simulink model "propagatorGuz_jupiter"  (R2024b)
settings: Solver=FixedStepAuto  StartTime=0.0  StopTime=tf  FixedStep=3600  MaxStep=43200  MinStep=3600  RelTol=1e-8  AbsTol=1e-8
undefined symbols (not defined in the file or in its folder): area, burnOverride, initMass, mDot, ref, thrust, thrustingThreshold, thrustingThresholdMn
libraries: vrlib x5, simulink x4, matrix_library x4, aerolibsatdyn x1, aerolibutil x1
settings Model: Creator=miqui  LastModifiedBy=benit
settings SolverCC: InitialStep=3600
settings RTWCC: GPUComputeCapability=3.5

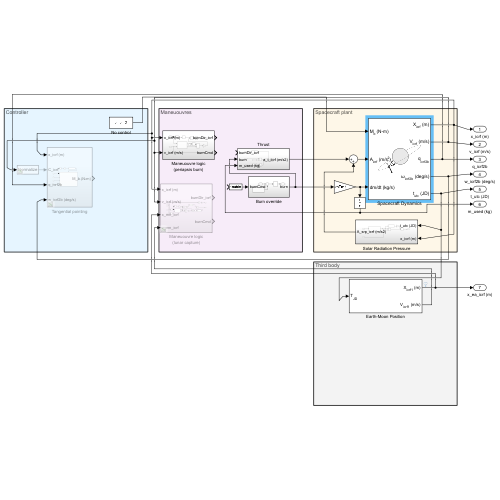
[thumbnail: Simulink's stored preview of the top-level diagram]
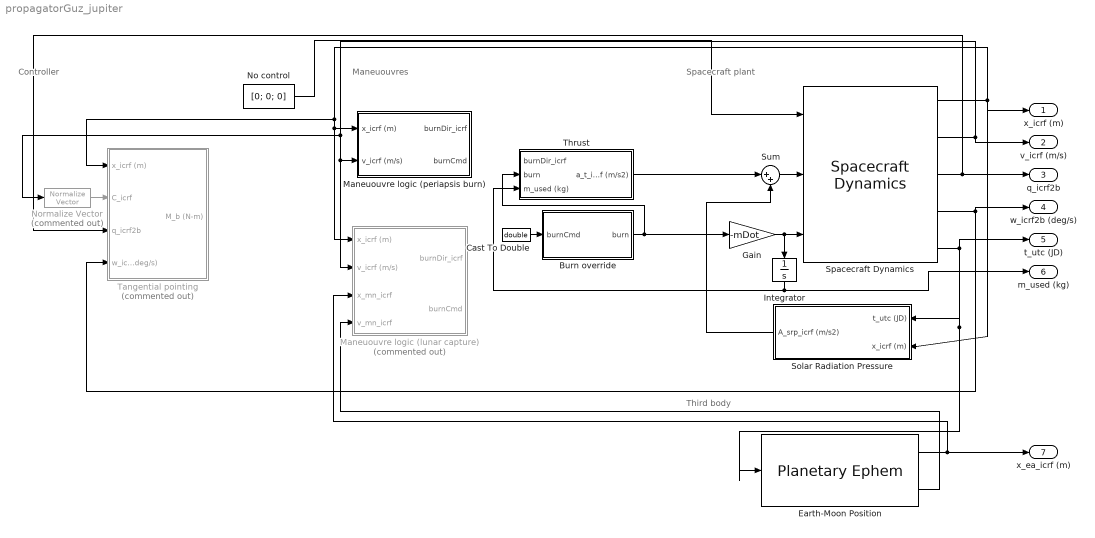
== system propagatorGuz_jupiter ==
  note: Third body
  note: Controller
  note: Maneuouvres
  note: Spacecraft plant
  Burn override : Subsystem
  Cast To Double : DataTypeConversion  OutDataTypeStr=double  SaturateOnIntegerOverflow=off  RndMeth=Floor
  Earth-Moon Position : PlanetaryEphem  units=m,m/s  center=Sun  target=Jupiter  useDateRange=on  startDate=startDate2  endDate=endDate
  Gain : Gain  Gain=-mDot
  Integrator : Integrator
  Maneuouvre logic (lunar capture) : Subsystem  Commented=on
  Maneuouvre logic (periapsis burn) : Subsystem
  No control : Constant  Value=[0; 0; 0]
  Normalize Vector : vrlib/Utilities/Normalize Vector  Commented=on  maxzero=0
  Solar Radiation Pressure : Subsystem
  Spacecraft Dynamics : SpacecraftDynamics  forcesIn=off  accelIn=on  startDate=startDate2  massType=Simple variable  mass=initMass  emptyMass=endMass  fullMass=initMass  inertia=[1, 0, 0; 0, 1, 0; 0, 0, 1]*initMass  outputFuelStatus=off  semiMajorAxis=sma  eccentricity=ecc  inclination=inc  raan=RAAN  argPeriapsis=aop  trueAnomaly=true_an  useGravGrad=off  centralBody=Sun  gravityModel=Point-mass  useEOPs=off  ephemerisStartDate=startDate2  ephemerisEndDate=endDate  useThirdBodyGravity=on  includeEarthGravity=off  includeMoonGravity=off  reflectivityCoeff=ref  srpArea=area
  Sum : Sum  Inputs=|++
  Tangential pointing : Subsystem  Commented=on
  Thrust : Subsystem
  x_icrf (m) : Outport
  v_icrf (m/s) : Outport  Port=2
  q_icrf2b : Outport  Port=3
  w_icrf2b (deg/s) : Outport  Port=4
  t_utc (JD) : Outport  Port=5
  m_used (kg) : Outport  Port=6
  x_ea_icrf (m) : Outport  Port=7
  wires:
  Spacecraft Dynamics/1 -> Maneuouvre logic (lunar capture)/1(x_icrf (m)), Maneuouvre logic (periapsis burn)/1(x_icrf (m)), Tangential pointing/1(x_icrf (m)), Solar Radiation Pressure/2(x_icrf (m)), x_icrf (m)/1
  Spacecraft Dynamics/2 -> Maneuouvre logic (lunar capture)/2(v_icrf (m/s)), Maneuouvre logic (periapsis burn)/2(v_icrf (m/s)), Normalize Vector/1, v_icrf (m/s)/1
  Spacecraft Dynamics/3 -> Tangential pointing/3(q_icrf2b), q_icrf2b/1
  Spacecraft Dynamics/4 -> Tangential pointing/4(w_icrf2b (deg/s)), w_icrf2b (deg/s)/1
  Spacecraft Dynamics/5 -> Earth-Moon Position/1, Solar Radiation Pressure/1(t_utc (JD)), t_utc (JD)/1
  Integrator/1 -> Thrust/3(m_used (kg)), m_used (kg)/1
  Gain/1 -> Spacecraft Dynamics/3, Integrator/1
  Sum/1 -> Spacecraft Dynamics/2
  Cast To Double/1 -> Burn override/1(burnCmd)
  Burn override/1(burn) -> Thrust/2(burn), Gain/1
  Thrust/1(a_t_icrf (m/s2)) -> Sum/1
  Earth-Moon Position/1 -> Maneuouvre logic (lunar capture)/3(x_mn_icrf), x_ea_icrf (m)/1
  Earth-Moon Position/2 -> Maneuouvre logic (lunar capture)/4(v_mn_icrf)
  Normalize Vector/1 -> Tangential pointing/2(C_icrf)
  No control/1 -> Spacecraft Dynamics/1
  Solar Radiation Pressure/1(A_srp_icrf (m/s2)) -> Sum/2

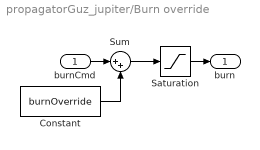
== system propagatorGuz_jupiter/Burn override ==
  burnCmd : Inport
  Constant : Constant  Value=burnOverride
  Saturation : Saturate  UpperLimit=1  LowerLimit=0
  Sum : Sum  Inputs=|++
  burn : Outport
  wires:
  Constant/1 -> Sum/2
  Saturation/1 -> burn/1
  burnCmd/1 -> Sum/1
  Sum/1 -> Saturation/1

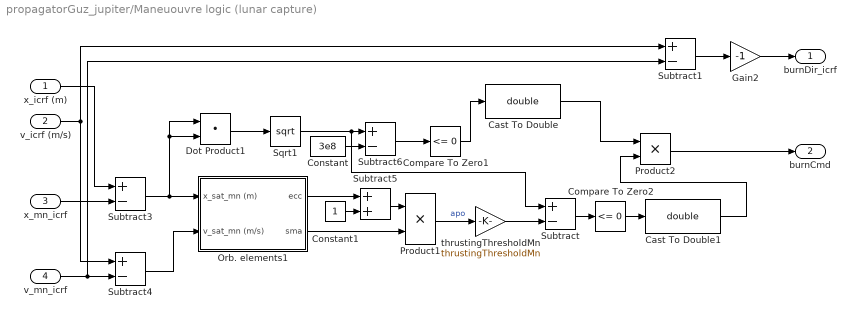
== system propagatorGuz_jupiter/Maneuouvre logic (lunar capture) ==
  x_icrf (m) : Inport
  v_icrf (m/s) : Inport  Port=2
  x_mn_icrf : Inport  Port=3
  v_mn_icrf : Inport  Port=4
  Cast To Double : DataTypeConversion  OutDataTypeStr=double  SaturateOnIntegerOverflow=off  RndMeth=Floor
  Cast To Double1 : DataTypeConversion  OutDataTypeStr=double  SaturateOnIntegerOverflow=off  RndMeth=Floor
  Compare To Zero1 : simulink/Logic and Bit Operations/Compare To Zero  relop=<=  OutDataTypeStr=boolean
  Compare To Zero2 : simulink/Logic and Bit Operations/Compare To Zero  relop=<=  OutDataTypeStr=boolean
  Constant : Constant  Value=3e8
  Constant1 : Constant
  Dot Product1 : DotProduct  OutDataTypeStr=Inherit: Inherit via internal rule
  Gain2 : Gain  Gain=-1
  Orb. elements1 : Subsystem
  Product1 : Product
  Product2 : Product
  Sqrt1 : Sqrt
  Subtract{,1,3..4,6} (5 alike) : Sum  Inputs=+-
  Subtract5 : Sum
  thrustingThresholdMn : Gain  Gain=thrustingThresholdMn
  burnDir_icrf : Outport
  burnCmd : Outport  Port=2
  wires:
  x_icrf (m)/1 -> Subtract3/1
  v_icrf (m/s)/1 -> Subtract1/1, Subtract4/1
  x_mn_icrf/1 -> Subtract3/2
  v_mn_icrf/1 -> Subtract4/2, Subtract1/2
  Subtract4/1 -> Orb. elements1/2(v_sat_mn (m/s))
  Subtract3/1 -> Dot Product1/1, Dot Product1/2, Orb. elements1/1(x_sat_mn (m))
  Subtract5/1 -> Product1/1
  Orb. elements1/2(sma) -> Product1/2
  Constant1/1 -> Subtract5/2
  Orb. elements1/1(ecc) -> Subtract5/1
  Subtract6/1 -> Compare To Zero1/1
  Dot Product1/1 -> Sqrt1/1
  Sqrt1/1 -> Subtract/1, Subtract6/1
  Compare To Zero1/1 -> Cast To Double/1
  Constant/1 -> Subtract6/2
  Product1/1 -> thrustingThresholdMn/1  "apo"
  thrustingThresholdMn/1 -> Subtract/2
  Subtract/1 -> Compare To Zero2/1
  Compare To Zero2/1 -> Cast To Double1/1
  Cast To Double1/1 -> Product2/2
  Cast To Double/1 -> Product2/1
  Product2/1 -> burnCmd/1
  Subtract1/1 -> Gain2/1
  Gain2/1 -> burnDir_icrf/1

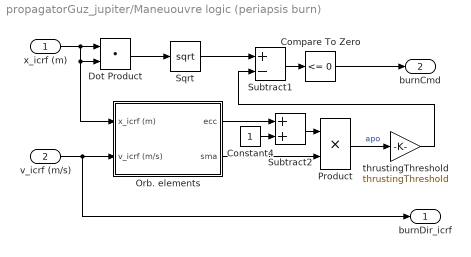
== system propagatorGuz_jupiter/Maneuouvre logic (periapsis burn) ==
  x_icrf (m) : Inport
  v_icrf (m/s) : Inport  Port=2
  Compare To Zero : simulink/Logic and Bit Operations/Compare To Zero  relop=<=  OutDataTypeStr=boolean
  Constant4 : Constant
  Dot Product : DotProduct  OutDataTypeStr=Inherit: Inherit via internal rule
  Orb. elements : Subsystem
  Product : Product
  Sqrt : Sqrt
  Subtract1 : Sum  Inputs=+-
  Subtract2 : Sum
  thrustingThreshold : Gain  Gain=thrustingThreshold
  burnDir_icrf : Outport
  burnCmd : Outport  Port=2
  wires:
  x_icrf (m)/1 -> Orb. elements/1(x_icrf (m)), Dot Product/2, Dot Product/1
  Subtract2/1 -> Product/1
  Compare To Zero/1 -> burnCmd/1
  Product/1 -> thrustingThreshold/1  "apo"
  Orb. elements/2(sma) -> Product/2
  Dot Product/1 -> Sqrt/1
  Constant4/1 -> Subtract2/2
  Orb. elements/1(ecc) -> Subtract2/1
  thrustingThreshold/1 -> Subtract1/2
  Sqrt/1 -> Subtract1/1
  Subtract1/1 -> Compare To Zero/1
  v_icrf (m/s)/1 -> Orb. elements/2(v_icrf (m/s)), burnDir_icrf/1

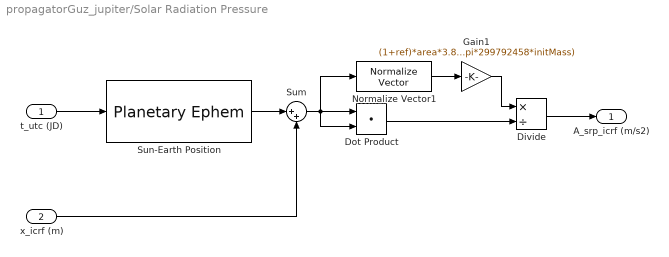
== system propagatorGuz_jupiter/Solar Radiation Pressure ==
  t_utc (JD) : Inport
  x_icrf (m) : Inport  Port=2
  Divide : Product  Inputs=*/
  Dot Product : DotProduct  OutDataTypeStr=Inherit: Inherit via internal rule
  Gain1 : Gain  Gain=(1+ref)*area*3.852e26/(4*pi*299792458*initMass)
  Normalize Vector1 : vrlib/Utilities/Normalize Vector  maxzero=0
  Sum : Sum  Inputs=|++
  Sun-Earth Position : PlanetaryEphem  units=m,m/s  center=Sun  target=Earth  outputVelocity=off
  A_srp_icrf (m/s2) : Outport
  wires:
  Normalize Vector1/1 -> Gain1/1
  Gain1/1 -> Divide/1
  Dot Product/1 -> Divide/2
  Divide/1 -> A_srp_icrf (m/s2)/1
  t_utc (JD)/1 -> Sun-Earth Position/1
  Sun-Earth Position/1 -> Sum/1
  Sum/1 -> Dot Product/1, Normalize Vector1/1, Dot Product/2
  x_icrf (m)/1 -> Sum/2

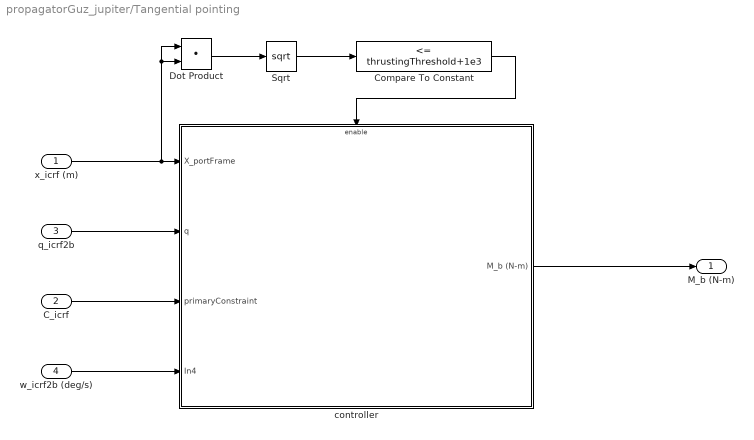
== system propagatorGuz_jupiter/Tangential pointing ==
  x_icrf (m) : Inport
  C_icrf : Inport  Port=2
  q_icrf2b : Inport  Port=3
  w_icrf2b (deg/s) : Inport  Port=4
  Compare To Constant : simulink/Logic and Bit Operations/Compare To Constant  relop=<=  const=thrustingThreshold+1e3  OutDataTypeStr=boolean
  Dot Product : DotProduct  OutDataTypeStr=Inherit: Inherit via internal rule
  Sqrt : Sqrt
  controller : Subsystem
  M_b (N-m) : Outport
  wires:
  q_icrf2b/1 -> controller/2(q)
  C_icrf/1 -> controller/3(primaryConstraint)
  w_icrf2b (deg/s)/1 -> controller/4(In4)
  controller/1(M_b (N-m)) -> M_b (N-m)/1
  Dot Product/1 -> Sqrt/1
  Sqrt/1 -> Compare To Constant/1
  x_icrf (m)/1 -> Dot Product/1, Dot Product/2, controller/1(X_portFrame)
  Compare To Constant/1 -> controller/Enable

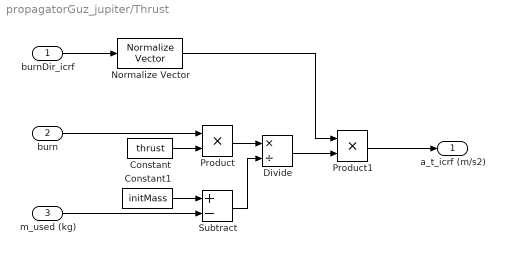
== system propagatorGuz_jupiter/Thrust ==
  burnDir_icrf : Inport
  burn : Inport  Port=2
  m_used (kg) : Inport  Port=3
  Constant : Constant  Value=thrust
  Constant1 : Constant  Value=initMass
  Divide : Product  Inputs=*/
  Normalize Vector : vrlib/Utilities/Normalize Vector  maxzero=0
  Product : Product
  Product1 : Product
  Subtract : Sum  Inputs=+-
  a_t_icrf (m/s2) : Outport
  wires:
  burn/1 -> Product/1
  Constant/1 -> Product/2
  Product/1 -> Divide/1
  Constant1/1 -> Subtract/1
  m_used (kg)/1 -> Subtract/2
  Subtract/1 -> Divide/2
  burnDir_icrf/1 -> Normalize Vector/1
  Product1/1 -> a_t_icrf (m/s2)/1
  Divide/1 -> Product1/2
  Normalize Vector/1 -> Product1/1

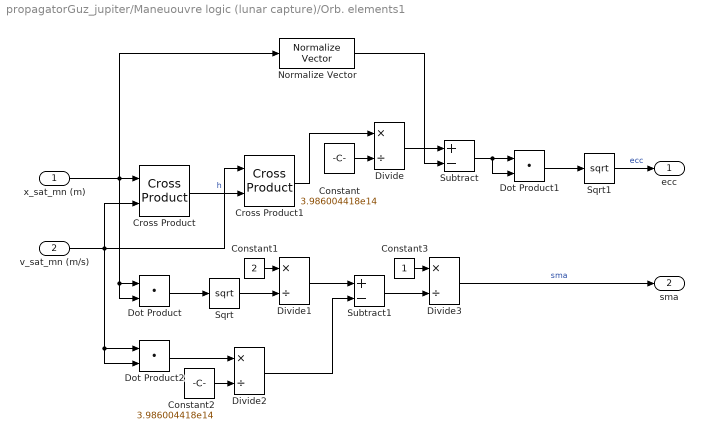
== system propagatorGuz_jupiter/Maneuouvre logic (lunar capture)/Orb. elements1 ==
  x_sat_mn (m) : Inport
  v_sat_mn (m/s) : Inport  Port=2
  Constant : Constant  Value=3.986004418e14
  Constant1 : Constant  Value=2
  Constant2 : Constant  Value=3.986004418e14
  Constant3 : Constant
  Cross Product : matrix_library/Cross Product
  Cross Product1 : matrix_library/Cross Product
  Divide{,1..3} (4 alike) : Product  Inputs=*/
  Dot Product : DotProduct  OutDataTypeStr=Inherit: Inherit via internal rule
  Dot Product1 : DotProduct  OutDataTypeStr=Inherit: Inherit via internal rule
  Dot Product2 : DotProduct  OutDataTypeStr=Inherit: Inherit via internal rule
  Normalize Vector : vrlib/Utilities/Normalize Vector  maxzero=0
  Sqrt : Sqrt
  Sqrt1 : Sqrt
  Subtract : Sum  Inputs=+-
  Subtract1 : Sum  Inputs=+-
  ecc : Outport
  sma : Outport  Port=2
  wires:
  x_sat_mn (m)/1 -> Normalize Vector/1, Dot Product/2, Dot Product/1, Cross Product/1
  v_sat_mn (m/s)/1 -> Dot Product2/2, Dot Product2/1, Cross Product1/1, Cross Product/2
  Cross Product/1 -> Cross Product1/2  "h"
  Constant/1 -> Divide/2
  Cross Product1/1 -> Divide/1
  Dot Product/1 -> Sqrt/1
  Sqrt/1 -> Divide1/2
  Divide/1 -> Subtract/1
  Normalize Vector/1 -> Subtract/2
  Dot Product1/1 -> Sqrt1/1
  Subtract/1 -> Dot Product1/2, Dot Product1/1
  Dot Product2/1 -> Divide2/1
  Constant1/1 -> Divide1/1
  Constant2/1 -> Divide2/2
  Divide1/1 -> Subtract1/1
  Divide2/1 -> Subtract1/2
  Subtract1/1 -> Divide3/2
  Constant3/1 -> Divide3/1
  Sqrt1/1 -> ecc/1  "ecc"
  Divide3/1 -> sma/1  "sma"

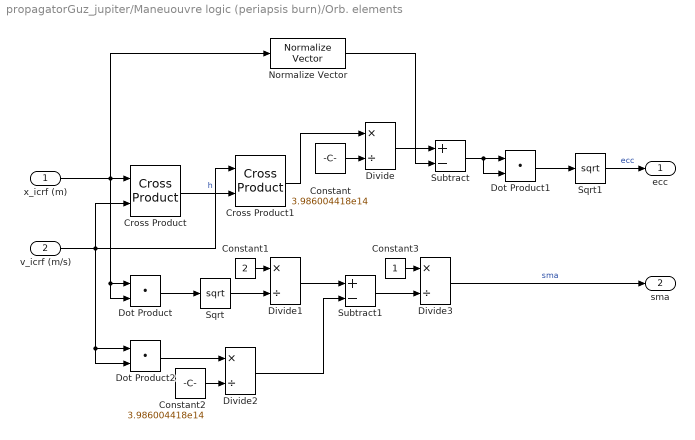
== system propagatorGuz_jupiter/Maneuouvre logic (periapsis burn)/Orb. elements ==
  x_icrf (m) : Inport
  v_icrf (m/s) : Inport  Port=2
  Constant : Constant  Value=3.986004418e14
  Constant1 : Constant  Value=2
  Constant2 : Constant  Value=3.986004418e14
  Constant3 : Constant
  Cross Product : matrix_library/Cross Product
  Cross Product1 : matrix_library/Cross Product
  Divide{,1..3} (4 alike) : Product  Inputs=*/
  Dot Product : DotProduct  OutDataTypeStr=Inherit: Inherit via internal rule
  Dot Product1 : DotProduct  OutDataTypeStr=Inherit: Inherit via internal rule
  Dot Product2 : DotProduct  OutDataTypeStr=Inherit: Inherit via internal rule
  Normalize Vector : vrlib/Utilities/Normalize Vector  maxzero=0
  Sqrt : Sqrt
  Sqrt1 : Sqrt
  Subtract : Sum  Inputs=+-
  Subtract1 : Sum  Inputs=+-
  ecc : Outport
  sma : Outport  Port=2
  wires:
  x_icrf (m)/1 -> Normalize Vector/1, Dot Product/2, Dot Product/1, Cross Product/1
  v_icrf (m/s)/1 -> Dot Product2/2, Dot Product2/1, Cross Product1/1, Cross Product/2
  Cross Product/1 -> Cross Product1/2  "h"
  Constant/1 -> Divide/2
  Cross Product1/1 -> Divide/1
  Dot Product/1 -> Sqrt/1
  Sqrt/1 -> Divide1/2
  Divide/1 -> Subtract/1
  Normalize Vector/1 -> Subtract/2
  Dot Product1/1 -> Sqrt1/1
  Subtract/1 -> Dot Product1/2, Dot Product1/1
  Dot Product2/1 -> Divide2/1
  Constant1/1 -> Divide1/1
  Constant2/1 -> Divide2/2
  Divide1/1 -> Subtract1/1
  Divide2/1 -> Subtract1/2
  Subtract1/1 -> Divide3/2
  Constant3/1 -> Divide3/1
  Sqrt1/1 -> ecc/1  "ecc"
  Divide3/1 -> sma/1  "sma"

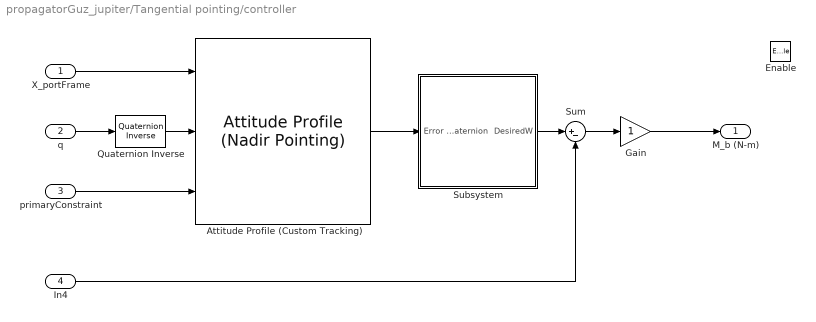
== system propagatorGuz_jupiter/Tangential pointing/controller ==
  X_portFrame : Inport
  q : Inport  Port=2
  primaryConstraint : Inport  Port=3
  In4 : Inport  Port=4
  Enable : EnablePort
  Attitude Profile (Custom Tracking) : aerolibsatdyn/Attitude Profile (Nadir Pointing)  outputError=on  outputFinalAttitude=off  portFrame=ICRF  pointingMode=Custom  celestialTarget=Sun  tunablePointing=off  primaryAlignmentSrc=Dialog  primaryAlignment=[1 0 0]  secondaryAlignmentSrc=Dialog  secondaryAlignment=[0 0 1]  constraintFrame=ICRF  primaryConstraintSrc=Port  primaryConstraint=[1 0 0]  secondaryConstraintSrc=Dialog  secondaryConstraint=[0 0 1]
      settings: LibrarySourceBlock=|
      | aerolibsatdyn/Attitude Profile
      | (Sun Tracking)
  Gain : Gain
  Quaternion Inverse : aerolibutil/Quaternion Inverse
  Subsystem : Subsystem
  Sum : Sum  Inputs=|+-
  M_b (N-m) : Outport
  wires:
  X_portFrame/1 -> Attitude Profile (Custom Tracking)/1
  Sum/1 -> Gain/1
  primaryConstraint/1 -> Attitude Profile (Custom Tracking)/3
  Quaternion Inverse/1 -> Attitude Profile (Custom Tracking)/2
  Attitude Profile (Custom Tracking)/1 -> Subsystem/1(Error quaternion)
  Gain/1 -> M_b (N-m)/1
  Subsystem/1(DesiredW) -> Sum/1
  In4/1 -> Sum/2
  q/1 -> Quaternion Inverse/1

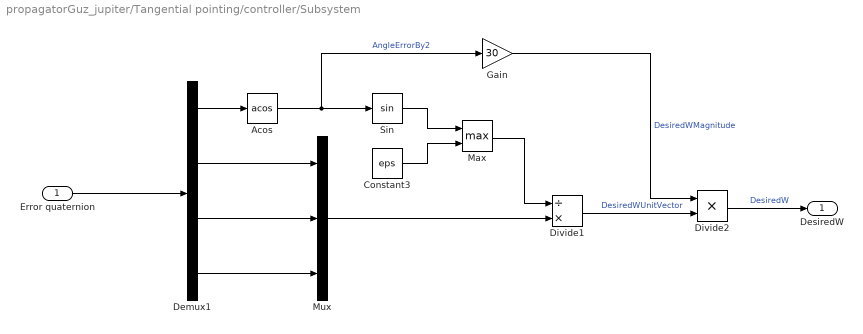
== system propagatorGuz_jupiter/Tangential pointing/controller/Subsystem ==
  Error quaternion : Inport
  Acos : Trigonometry  Operator=acos
  Constant3 : Constant  Value=eps
  Demux1 : Demux
  Divide1 : Product  Inputs=/*
  Divide2 : Product  Inputs=**
  Gain : Gain  Gain=30
  Max : MinMax  Function=max  Inputs=2
  Mux : Mux  Inputs=3
  Sin : Trigonometry
  DesiredW : Outport
  wires:
  Error quaternion/1 -> Demux1/1
  Gain/1 -> Divide2/1  "DesiredWMagnitude"
  Demux1/2 -> Mux/1
  Demux1/1 -> Acos/1
  Acos/1 -> Sin/1, Gain/1  "AngleErrorBy2"
  Mux/1 -> Divide1/2
  Divide2/1 -> DesiredW/1  "DesiredW"
  Constant3/1 -> Max/2
  Demux1/3 -> Mux/2
  Max/1 -> Divide1/1
  Demux1/4 -> Mux/3
  Sin/1 -> Max/1
  Divide1/1 -> Divide2/2  "DesiredWUnitVector"
